simulink model "Equivalente"  (R2023b)
settings: Solver=VariableStepAuto  StartTime=0.0  StopTime=10.0  RelTol=1e-3
values from neighbouring files (symbols this model uses):
  Cts = 0.818    [parametros_proyecto2.m]
  Lq = 5.8e-3    (= 0.0058)    [parametros_proyecto2.m]
  Rs_ref = 1.02    [parametros_proyecto2.m]
  Rts_amb = 146.7    [parametros_proyecto2.m]
undefined symbols (not defined in the file or in its folder): magnitude, P_p
settings Model: Creator=ignab  LastModifiedBy=ignab

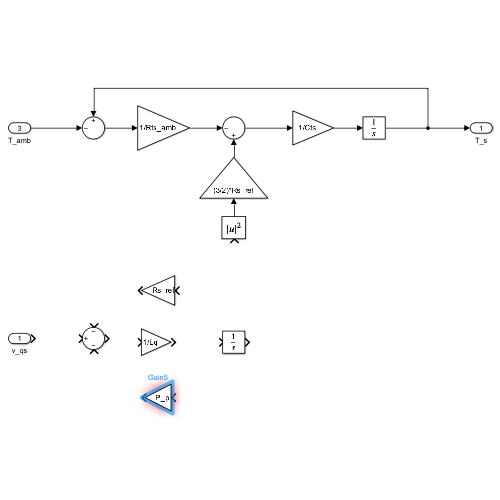
[thumbnail: Simulink's stored preview of the top-level diagram]
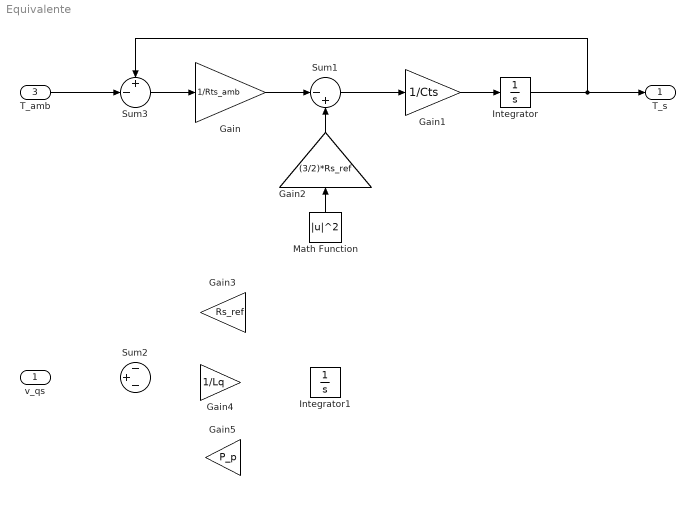
== system Equivalente ==
  v_qs : Inport
  T_amb : Inport  Port=3
  Gain : Gain  Gain=1/Rts_amb
  Gain1 : Gain  Gain=1/Cts
  Gain2 : Gain  Gain=(3/2)*Rs_ref
  Gain3 : Gain  Gain=Rs_ref
  Gain4 : Gain  Gain=1/Lq
  Gain5 : Gain  Gain=P_p
  Integrator : Integrator
  Integrator1 : Integrator
  Math Function : Math  Operator=magnitude^2
  Sum1 : Sum  Inputs=|-+
  Sum2 : Sum  Inputs=-+-
  Sum3 : Sum  Inputs=+-|
  T_s : Outport
  wires:
  T_amb/1 -> Sum3/2
  Sum3/1 -> Gain/1
  Gain2/1 -> Sum1/2
  Gain/1 -> Sum1/1
  Sum1/1 -> Gain1/1
  Gain1/1 -> Integrator/1
  Integrator/1 -> Sum3/1, T_s/1
  Math Function/1 -> Gain2/1
